simulink model "V_F spwm"  (R2023a)
settings: Solver=ode23tb  StartTime=0.0  StopTime=5  MaxStep=1e-4  RelTol=1e-3
libraries: spsIGBTDiodeLib x6, spsSawtoothGeneratorLib x3, spsAsynchronousMachineSIUnitsLib x1, spsDCVoltageSourceLib x1, simulink x1, spsVoltageMeasurementLib x1, sps_lib x1
settings Model: Creator=dell  LastModifiedBy=dell

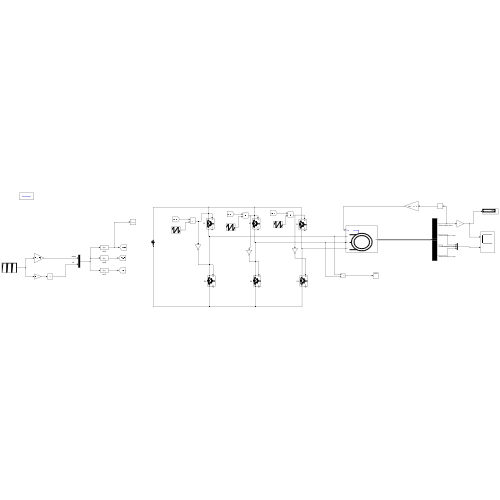
[thumbnail: Simulink's stored preview of the top-level diagram]
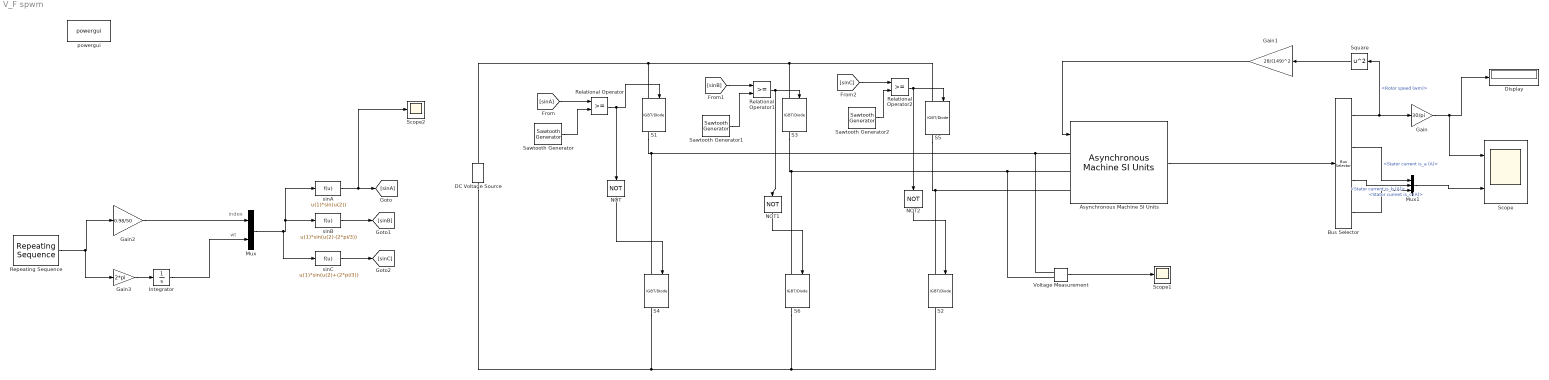
== system V_F spwm ==
  note: wt
  note: index
  Asynchronous Machine SI Units : spsAsynchronousMachineSIUnitsLib/Asynchronous Machine SI Units  RotorType=Squirrel-cage  PresetModel="15:  5.4 HP (4KW)   400 V  50Hz 1430 RPM"  MechanicalLoad=Torque Tm  ShowDetailedParameters=on  ReferenceFrame=Rotor  Units=SI  MeasurementBus=off  NominalParameters=[4000 400 50]  VoltageRatio=1  Stator=[1.405 0.005839]  Rotor=[1.395 0.005839]  Cage1=[0.4155 0.002066]  Cage2=[0.4168 0.0003495]  Lm=0.1722  Mechanical=[0.0131 0.002985 2]  PolePairs=2  InitialConditions=[0 0 0 0 0 0 0 0]  SimulateSaturation=off  Saturation=[14.03593122, 27.81365428, 53.79336849, 72.68890987, 97.98006896, 148.6815601, 215.7428561, 302.9841135, 428.7778367 ; 230, 322, 414, 460, 506, 552, 598, 644, 690]  LoadFlowParameters=1492000  TsPowergui=0  TsBlock=-1  IterativeModel=Trapezoidal non iterative  IterativeDiscreteModel=Trapezoidal non iterative  Pmec=1.492e+006
  Bus Selector : BusSelector  OutputSignals=Mechanical.Rotor speed (wm),Stator measurements.Stator current is_a (A),Stator measurements.Stator current is_b (A),Stator measurements.Stator current is_c (A)
  DC Voltage Source : spsDCVoltageSourceLib/DC Voltage Source  Amplitude=650  Measurements=None
  Display : Display
  Gain : Gain  Gain=30/pi
  Gain1 : Gain  Gain=28/(149)^2
  Gain2 : Gain  Gain=0.98/50
  Gain3 : Gain  Gain=2*pi
  Integrator : Integrator
  Mux : Mux  Inputs=2
  Mux1 : Mux  Inputs=3
  NOT : Logic  Operator=NOT  IconShape=distinctive  AllPortsSameDT=off  OutDataTypeStr=boolean
  NOT1 : Logic  Operator=NOT  IconShape=distinctive  AllPortsSameDT=off  OutDataTypeStr=boolean
  NOT2 : Logic  Operator=NOT  IconShape=distinctive  AllPortsSameDT=off  OutDataTypeStr=boolean
  Relational Operator : RelationalOperator  OutDataTypeStr=boolean  RndMeth=Simplest  InputSameDT=off
  Relational Operator1 : RelationalOperator  OutDataTypeStr=boolean  RndMeth=Simplest  InputSameDT=off
  Relational Operator2 : RelationalOperator  OutDataTypeStr=boolean  RndMeth=Simplest  InputSameDT=off
  Repeating Sequence : simulink/Sources/Repeating Sequence  rep_seq_t=[0 2 10]  rep_seq_y=[0 50 50]
  S{1..6} (6 alike) : spsIGBTDiodeLib/IGBT//Diode  Ron=1e-3  Rs=1e5  Cs=inf  Measurements=on
  Sawtooth Generator : spsSawtoothGeneratorLib/Sawtooth Generator  Freq=1000  Phase=180  Ts=0
  Sawtooth Generator1 : spsSawtoothGeneratorLib/Sawtooth Generator  Freq=1000  Phase=180  Ts=0
  Sawtooth Generator2 : spsSawtoothGeneratorLib/Sawtooth Generator  Freq=1000  Phase=180  Ts=0
  Scope : Scope  NumInputPorts=2
  Scope1 : Scope
  Scope2 : Scope
  Square : Math  Operator=square
  Voltage Measurement : spsVoltageMeasurementLib/Voltage Measurement  PhasorSimulation=off  OutputType=Complex  PSBequivalent=0
  powergui : sps_lib/powergui  Priority=1  SimulationMode=Continuous  SampleTime=50e-6  frequency=60  Iterations=50  frequencyindice=0  Pbase=100e6  ErrMax=1e-4  UnitsV=kV  UnitsW=MW  buscounter=0  FunctionMessages=off  echomessages=off  EnableUseOfTLC=off  CurrentSourceSwitches=off  DisableSnubberDevices=off  DisableRonSwitches=off  DisableVfSwitches=off  DisplayEquations=off  AutomaticDiscreteSolvers=off  SolverType=Tustin/Backward Euler (TBE)  Interpol=off  ExternalGateDelay=off  methode=off  Ts=100  x0status=blocks  SPID=on  SwTol=0  HookPort=off  NonlinearTolerance=1e-4  nMaxIteration=100  ContinueOnMaxIteration=off  RestoreLinks=warning  ResistiveCurrentMeasurement=off  Frange=[0:2:500]  Ylog=off  Xlog=on  ShowGrid=off  save=off  variable=ZData  structure=0  ZoomFFT=off  StartTime=0.0  cycles=1  DisplayStyle=1  fundamental=60  FreqAxis=off  MaxFrequency=1000  frequencyindicesteady=1  RmsSteady=1  display=off
  sinA : Fcn  Expr=u(1)*sin(u(2))
  sinB : Fcn  Expr=u(1)*sin(u(2)-(2*pi/3))
  sinC : Fcn  Expr=u(1)*sin(u(2)+(2*pi/3))
  wires:
  Relational Operator2/1 -> S5/1, NOT2/1
  NOT1/1 -> S6/1
  Sawtooth Generator/1 -> Relational Operator/2
  NOT2/1 -> S2/1
  Sawtooth Generator2/1 -> Relational Operator2/2
  NOT/1 -> S4/1
  Sawtooth Generator1/1 -> Relational Operator1/2
  Relational Operator1/1 -> S3/1, NOT1/1
  Relational Operator/1 -> S1/1, NOT/1
  Asynchronous Machine SI Units/1 -> Bus Selector/1
  Bus Selector/1 -> Square/1, Gain/1  "<Rotor speed (wm)>"
  Gain/1 -> Scope/1, Display/1
  Square/1 -> Gain1/1
  Gain1/1 -> Asynchronous Machine SI Units/1
  Gain2/1 -> Mux/1
  Mux/1 -> sinC/1, sinB/1, sinA/1
  Gain3/1 -> Integrator/1
  Integrator/1 -> Mux/2
  Repeating Sequence/1 -> Gain3/1, Gain2/1
  sinA/1 -> Scope2/1, [sinA]
  sinB/1 -> [sinB]
  sinC/1 -> [sinC]
  [sinA] -> Relational Operator/1
  [sinB] -> Relational Operator1/1
  [sinC] -> Relational Operator2/1
  Voltage Measurement/1 -> Scope1/1
  Bus Selector/2 -> Mux1/1  "<Stator current is_a (A)>"
  Bus Selector/3 -> Mux1/2  "<Stator current is_b (A)>"
  Bus Selector/4 -> Mux1/3  "<Stator current is_c (A)>"
  Mux1/1 -> Scope/2
  connections:
  DC Voltage Source/RConn1 -- S1/LConn1 -- S3/LConn1 -- S5/LConn1
  S6/RConn1 -- S2/RConn1 -- S4/RConn1 -- DC Voltage Source/LConn1
  S1/RConn1 -- Voltage Measurement/LConn1 -- Asynchronous Machine SI Units/LConn1 -- S4/LConn1
  S3/RConn1 -- Voltage Measurement/LConn2 -- Asynchronous Machine SI Units/LConn2 -- S6/LConn1
  S5/RConn1 -- Asynchronous Machine SI Units/LConn3 -- S2/LConn1
